simulink model "Flight_Physics__ForStudent"  (R2017b)
settings: configuration reference "cs" (kept outside this file)
undefined symbols (not defined in the file or in its folder): Actuators, AeroDerivatives, Configuration, Engine, g, magnitude, Sim_Control, Ts
libraries: aerolibatmos2 x1
settings Model: Creator=zht  LastModifiedBy=ZHT
settings ConfigSetRef: SourceLocation=Base Workspace

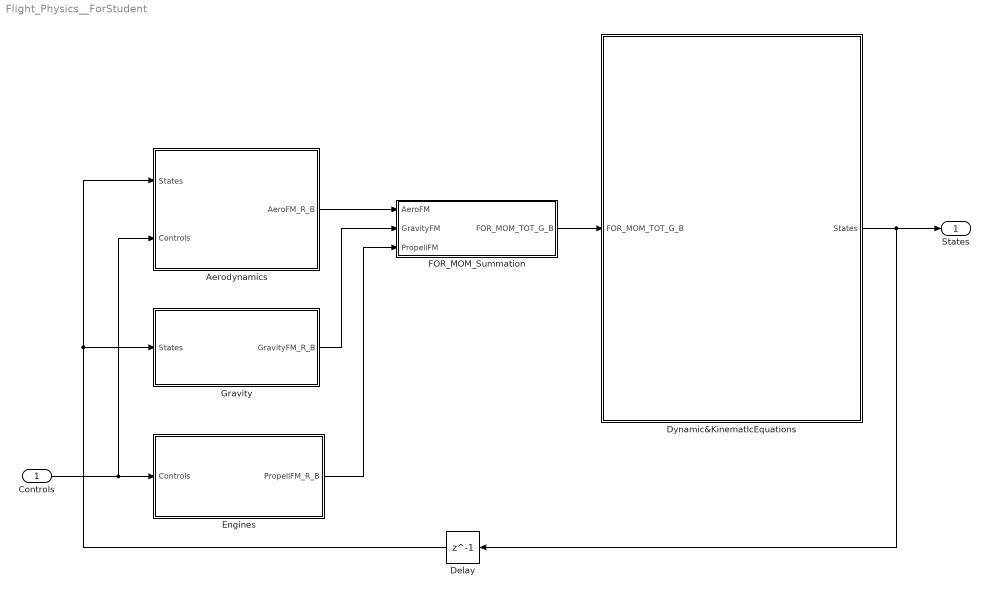
== system Flight_Physics__ForStudent ==
  Controls : Inport  OutDataTypeStr=Bus: Controls_CMD_BUS
  Aerodynamics : Subsystem
  Delay : Delay  DelayLength=1
  Dynamic&KinematlcEquations : Subsystem
  Engines : Subsystem
  FOR_MOM_Summation : Subsystem
  Gravity : Subsystem
  States : Outport  OutDataTypeStr=Bus: States_BUS
  wires:
  Controls/1 -> Engines/1(Controls), Aerodynamics/2(Controls)
  Dynamic&KinematlcEquations/1(States) -> States/1, Delay/1
  FOR_MOM_Summation/1(FOR_MOM_TOT_G_B) -> Dynamic&KinematlcEquations/1(FOR_MOM_TOT_G_B)
  Aerodynamics/1(AeroFM_R_B) -> FOR_MOM_Summation/1(AeroFM)
  Gravity/1(GravityFM_R_B) -> FOR_MOM_Summation/2(GravityFM)
  Engines/1(PropellFM_R_B) -> FOR_MOM_Summation/3(PropellFM)
  Delay/1 -> Aerodynamics/1(States), Gravity/1(States)

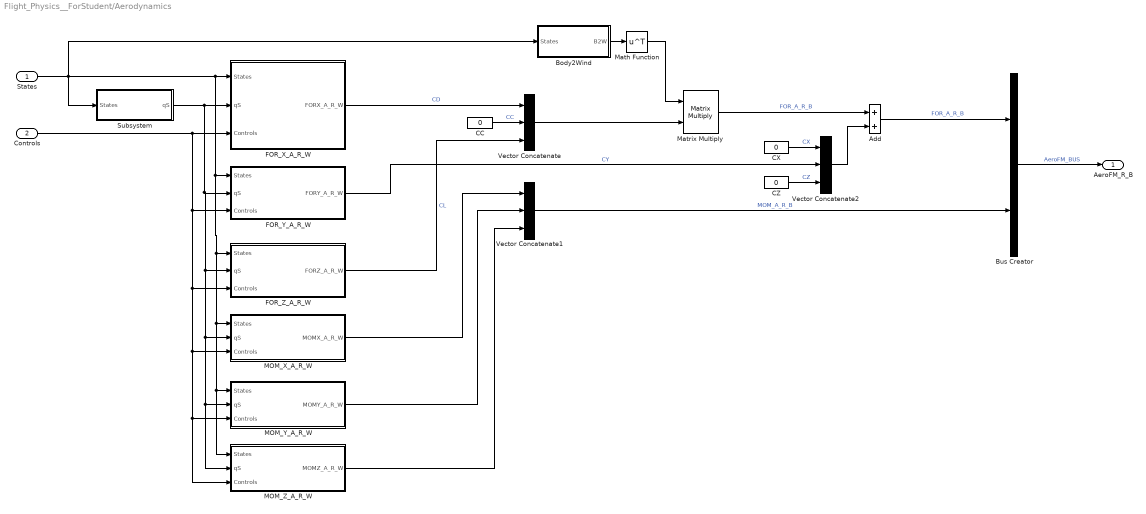
== system Flight_Physics__ForStudent/Aerodynamics ==
  States : Inport  OutDataTypeStr=Bus: States_BUS
  Controls : Inport  Port=2  OutDataTypeStr=Bus: Controls_CMD_BUS
  Add : Sum
  Body2Wind : Subsystem
  Bus Creator : BusCreator  Inputs=2  OutDataTypeStr=Bus: AeroFM_BUS
  CC : Constant  Value=0
  CX : Constant  Value=0
  CZ : Constant  Value=0
  FOR_X_A_R_W : Subsystem
  FOR_Y_A_R_W : Subsystem
  FOR_Z_A_R_W : Subsystem
  MOM_X_A_R_W : Subsystem
  MOM_Y_A_R_W : Subsystem
  MOM_Z_A_R_W : Subsystem
  Math Function : Math  Operator=transpose  SaturateOnIntegerOverflow=on
  Matrix Multiply : Product  Multiplication=Matrix(*)
  Subsystem : Subsystem
  Vector Concatenate : Concatenate  NumInputs=3  Mode=Multidimensional array
  Vector Concatenate1 : Concatenate  NumInputs=3  Mode=Multidimensional array
  Vector Concatenate2 : Concatenate  NumInputs=3  Mode=Multidimensional array
  AeroFM_R_B : Outport  OutDataTypeStr=Bus: AeroFM_BUS
  wires:
  Math Function/1 -> Matrix Multiply/1
  Add/1 -> Bus Creator/1  "FOR_A_R_B"
  Vector Concatenate1/1 -> Bus Creator/2  "MOM_A_R_B"
  MOM_Y_A_R_W/1(MOMY_A_R_W) -> Vector Concatenate1/2
  FOR_Z_A_R_W/1(FORZ_A_R_W) -> Vector Concatenate/3  "CL"
  FOR_Y_A_R_W/1(FORY_A_R_W) -> Vector Concatenate2/2  "CY"
  Body2Wind/1(B2W) -> Math Function/1
  Controls/1 -> FOR_Y_A_R_W/3(Controls), FOR_Z_A_R_W/3(Controls), MOM_X_A_R_W/3(Controls), MOM_Y_A_R_W/3(Controls), MOM_Z_A_R_W/3(Controls), FOR_X_A_R_W/3(Controls)
  Subsystem/1(qS) -> FOR_Z_A_R_W/2(qS), MOM_X_A_R_W/2(qS), MOM_Y_A_R_W/2(qS), MOM_Z_A_R_W/2(qS), FOR_Y_A_R_W/2(qS), FOR_X_A_R_W/2(qS)
  MOM_Z_A_R_W/1(MOMZ_A_R_W) -> Vector Concatenate1/3
  Bus Creator/1 -> AeroFM_R_B/1  "AeroFM_BUS"
  States/1 -> Subsystem/1(States), Body2Wind/1(States), MOM_Z_A_R_W/1(States), MOM_Y_A_R_W/1(States), MOM_X_A_R_W/1(States), FOR_Z_A_R_W/1(States), FOR_Y_A_R_W/1(States), FOR_X_A_R_W/1(States)
  MOM_X_A_R_W/1(MOMX_A_R_W) -> Vector Concatenate1/1
  FOR_X_A_R_W/1(FORX_A_R_W) -> Vector Concatenate/1  "CD"
  Vector Concatenate/1 -> Matrix Multiply/2
  CC/1 -> Vector Concatenate/2  "CC"
  CX/1 -> Vector Concatenate2/1  "CX"
  CZ/1 -> Vector Concatenate2/3  "CZ"
  Matrix Multiply/1 -> Add/1  "FOR_A_R_B"
  Vector Concatenate2/1 -> Add/2

== system Flight_Physics__ForStudent/Dynamic&KinematlcEquations ==
  note: 建模符号约定：
      | 变量命名：
      | 变量_运动类型_点_坐标系
      |
      | 变量类型：
      | VEL 速度（3x1的向量）
      | ROT 角速度（3x1的向量）
      | POS 位置（3x1的向量）
      | ATT 角度（3x1的向量）
      | VEL _DOT 加速度（3x1的向量）
      | ROT_DOT 角加速度（3x1的向量）
      | Alpha 迎角
      | Beta 侧滑角
      | Gamma 航迹倾角（下滑角、爬升角）
      | 运动类型：
      | K 表示相对于地面的运动
      | A 表示相对于气流的运动（考虑风场）
      | 点类型：
      | R 表示参考重心
      | G 表示实际重心
      | 坐标系类型：
      | B 机体系
      | E 地面系 ABS 与坐标系无关，表示该变量的绝对值
  FOR_MOM_TOT_G_B : Inport  OutDataTypeStr=Bus: FOR_MOM_TOT_BUS
  Bus Creator1 : BusCreator  Inputs=14  OutDataTypeStr=Bus: States_BUS
  Bus Selector1 : BusSelector  OutputSignals=FOR_T_G_B,MOM_T_G_B
  Bus Selector2 : BusSelector  OutputSignals=VEL_K_R_B,ROT_K_R_B,ATT_EULER
  Equations : Subsystem
  States : Outport  OutDataTypeStr=Bus: States_BUS
  wires:
  Bus Selector2/2 -> Equations/4(p_q_r)  "<ROT_K_R_B>"
  Bus Selector2/1 -> Equations/3(ub_vb_wb)  "<VEL_K_R_B>"
  Bus Selector2/3 -> Equations/5(phi_theta_psi)  "<ATT_EULER>"
  Equations/7(ROT_DOT_K_R_B) -> Bus Creator1/7  "ROT_DOT_K_R_B"
  Equations/10(VEL_K_R_ABS) -> Bus Creator1/10  "VEL_K_R_ABS"
  Bus Selector1/1 -> Equations/1(Fxyz(N))  "<FOR_T_G_B>"
  Equations/14(Beta_A_R_B) -> Bus Creator1/14  "Beta_A_R_B"
  Equations/12(Gamma_K_R_B) -> Bus Creator1/12  "Gamma_K_R_B"
  Equations/6(ROT_K_R_B) -> Bus Creator1/6  "ROT_K_R_B"
  Equations/13(Alpha_A_R_B) -> Bus Creator1/13  "Alpha_A_R_B"
  Equations/8(VEL_DOT_K_R_B) -> Bus Creator1/8  "VEL_DOT_K_R_B"
  Equations/5(VEL_K_R_B) -> Bus Creator1/5  "VEL_K_R_B"
  Equations/2(POS_R_E) -> Bus Creator1/2  "POS_R_E"
  Bus Creator1/1 -> Bus Selector2/1, States/1
  Bus Selector1/2 -> Equations/2(Mxyz(Nm))  "<MOM_T_G_B>"
  Equations/11(Chi_K_R_B) -> Bus Creator1/11  "Chi_K_R_B"
  Equations/1(VEL_K_R_E) -> Bus Creator1/1  "VEL_K_R_E"
  FOR_MOM_TOT_G_B/1 -> Bus Selector1/1
  Equations/9(FUEL_Availible) -> Bus Creator1/9  "FUEL_Availible"
  Equations/3(ATT_EULER) -> Bus Creator1/3  "ATT_EULER"
  Equations/4(M_BE) -> Bus Creator1/4  "M_BE"

== system Flight_Physics__ForStudent/Engines ==
  Controls : Inport  OutDataTypeStr=Bus: Controls_CMD_BUS
  1-D Lookup Table : Lookup_n-D  NumberOfTableDimensions=1  BreakpointsForDimension1=Engine.Thrset  Table=Engine.Tset  InternalRulePriority=Speed  RndMeth=Simplest  InputSameDT=on
  1-D Lookup Table1 : Lookup_n-D  NumberOfTableDimensions=1  BreakpointsForDimension1=Engine.Thrset  Table=Engine.SFCset  InternalRulePriority=Speed  RndMeth=Simplest  InputSameDT=on
  Bus Creator : BusCreator  Inputs=3  OutDataTypeStr=Bus: PropellFM_BUS
  Bus Selector : BusSelector  OutputSignals=Engine_CMD
  Constant4 : Constant  Value=Engine.Position-Configuration.POS_CG  SampleTime=Ts
  Constant5 : Constant  Value=Engine.Phi  SampleTime=Ts
  Gain : Gain  Gain=[1,0,0]'
  Gain1 : Gain  Gain=100
  Matrix Multiply : Product  Multiplication=Matrix(*)
  Subsystem : Subsystem
  Subsystem1 : Subsystem
  PropellFM_R_B : Outport  OutDataTypeStr=Bus: PropellFM_BUS
  wires:
  1-D Lookup Table1/1 -> Bus Creator/3  "SFC"
  Subsystem/1(M_B_Phi) -> Matrix Multiply/1
  Matrix Multiply/1 -> Subsystem1/2(v2), Bus Creator/2  "FOR_P_R_B"
  Bus Creator/1 -> PropellFM_R_B/1  "PropellFM_BUS"
  Bus Selector/1 -> 1-D Lookup Table1/1, Gain1/1  "<Engine_CMD>"
  Gain1/1 -> 1-D Lookup Table/1
  1-D Lookup Table/1 -> Gain/1
  Constant4/1 -> Subsystem1/1(v1)
  Controls/1 -> Bus Selector/1
  Gain/1 -> Matrix Multiply/2
  Constant5/1 -> Subsystem/1(Phi_rad)
  Subsystem1/1(v1_x_v2) -> Bus Creator/1  "MOM_P_R_B"

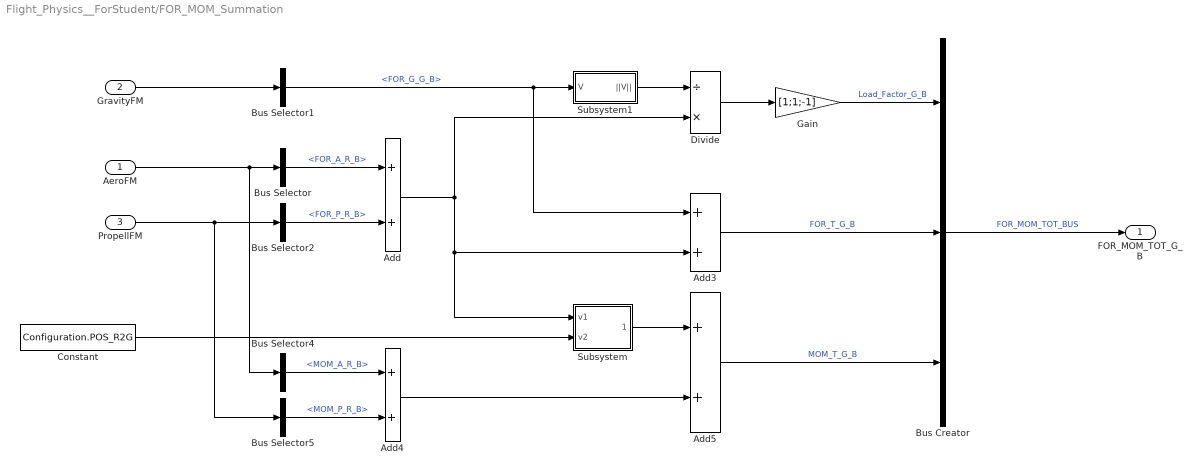
== system Flight_Physics__ForStudent/FOR_MOM_Summation ==
  AeroFM : Inport  OutDataTypeStr=Bus: AeroFM_BUS
  GravityFM : Inport  Port=2  OutDataTypeStr=Bus: GravityFM_BUS
  PropellFM : Inport  Port=3  OutDataTypeStr=Bus: PropellFM_BUS
  Add{,3..5} (4 alike) : Sum
  Bus Creator : BusCreator  Inputs=3  OutDataTypeStr=Bus: FOR_MOM_TOT_BUS
  Bus Selector : BusSelector  OutputSignals=FOR_A_R_B
  Bus Selector1 : BusSelector  OutputSignals=FOR_G_G_B
  Bus Selector2 : BusSelector  OutputSignals=FOR_P_R_B
  Bus Selector4 : BusSelector  OutputSignals=MOM_A_R_B
  Bus Selector5 : BusSelector  OutputSignals=MOM_P_R_B
  Constant : Constant  Value=Configuration.POS_R2G
  Divide : Product  Inputs=/*
  Gain : Gain  Gain=[1;1;-1]
  Subsystem : Subsystem
  Subsystem1 : Subsystem
  FOR_MOM_TOT_G_B : Outport  OutDataTypeStr=Bus: FOR_MOM_TOT_BUS
  wires:
  PropellFM/1 -> Bus Selector2/1, Bus Selector5/1
  AeroFM/1 -> Bus Selector4/1, Bus Selector/1
  GravityFM/1 -> Bus Selector1/1
  Bus Creator/1 -> FOR_MOM_TOT_G_B/1  "FOR_MOM_TOT_BUS"
  Bus Selector/1 -> Add/1  "<FOR_A_R_B>"
  Bus Selector2/1 -> Add/2  "<FOR_P_R_B>"
  Bus Selector1/1 -> Subsystem1/1(V), Add3/1  "<FOR_G_G_B>"
  Add/1 -> Subsystem/1(v1), Add3/2, Divide/2
  Subsystem1/1(||V||) -> Divide/1
  Divide/1 -> Gain/1
  Gain/1 -> Bus Creator/1  "Load_Factor_G_B"
  Add3/1 -> Bus Creator/2  "FOR_T_G_B"
  Bus Selector4/1 -> Add4/1  "<MOM_A_R_B>"
  Bus Selector5/1 -> Add4/2  "<MOM_P_R_B>"
  Subsystem/1(v1_x_v2) -> Add5/1
  Add4/1 -> Add5/2
  Add5/1 -> Bus Creator/3  "MOM_T_G_B"
  Constant/1 -> Subsystem/2(v2)

== system Flight_Physics__ForStudent/Gravity ==
  States : Inport  OutDataTypeStr=Bus: States_BUS
  Bus Creator : BusCreator  Inputs=2  OutDataTypeStr=Bus: GravityFM_BUS
  Bus Selector : BusSelector  OutputSignals=M_BE
  Constant : Constant  Value=[0;0;0]
  Constant1 : Constant  Value=[0;0;g]  SampleTime=Ts
  Constant2 : Constant  Value=Configuration.Mass  SampleTime=Ts
  Matrix Multiply : Product  Multiplication=Matrix(*)
  Product : Product
  GravityFM_R_B : Outport  OutDataTypeStr=Bus: GravityFM_BUS
  wires:
  States/1 -> Bus Selector/1
  Bus Selector/1 -> Matrix Multiply/1  "<M_BE>"
  Constant1/1 -> Matrix Multiply/2
  Matrix Multiply/1 -> Product/1
  Constant2/1 -> Product/2
  Product/1 -> Bus Creator/1  "FOR_G_G_B"
  Constant/1 -> Bus Creator/2  "MOM_G_G_B"
  Bus Creator/1 -> GravityFM_R_B/1  "GravityFM_BUS"

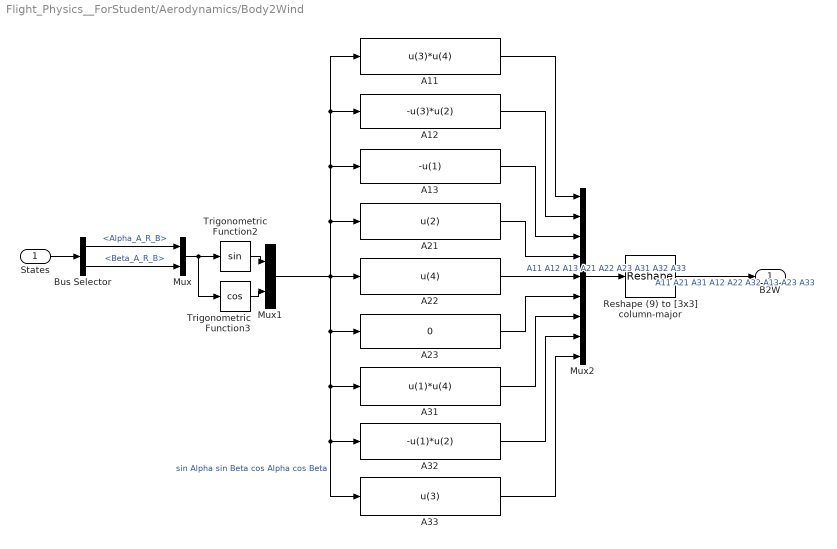
== system Flight_Physics__ForStudent/Aerodynamics/Body2Wind ==
  States : Inport  OutDataTypeStr=Bus: States_BUS
  A11 : Fcn  Expr=u(3)*u(4)
  A12 : Fcn  Expr=-u(3)*u(2)
  A13 : Fcn  Expr=-u(1)
  A21 : Fcn  Expr=u(2)
  A22 : Fcn  Expr=u(4)
  A23 : Fcn  Expr=0
  A31 : Fcn  Expr=u(1)*u(4)
  A32 : Fcn  Expr=-u(1)*u(2)
  A33 : Fcn  Expr=u(3)
  Bus Selector : BusSelector  OutputSignals=Alpha_A_R_B,Beta_A_R_B
  Mux : Mux  Inputs=2
  Mux1 : Mux  Inputs=2
  Mux2 : Mux  Inputs=9
  Reshape (9) to [3x3] column-major : Reshape  OutputDimensionality=Customize  OutputDimensions=[3,3]
  Trigonometric Function2 : Trigonometry
  Trigonometric Function3 : Trigonometry  Operator=cos
  B2W : Outport  PortDimensions=[3 3]
  wires:
  Mux/1 -> Trigonometric Function2/1, Trigonometric Function3/1
  Trigonometric Function3/1 -> Mux1/2
  Trigonometric Function2/1 -> Mux1/1
  Bus Selector/2 -> Mux/2  "<Beta_A_R_B>"
  Bus Selector/1 -> Mux/1  "<Alpha_A_R_B>"
  States/1 -> Bus Selector/1
  A12/1 -> Mux2/2
  A13/1 -> Mux2/3
  A21/1 -> Mux2/4
  A32/1 -> Mux2/8
  A23/1 -> Mux2/6
  Mux2/1 -> Reshape (9) to [3x3] column-major/1  "A11 A12 A13 A21 A22 A23 A31 A32 A33"
  Reshape (9) to [3x3] column-major/1 -> B2W/1  "A11 A21 A31 A12 A22 A32 A13 A23 A33"
  A11/1 -> Mux2/1
  A22/1 -> Mux2/5
  A33/1 -> Mux2/9
  Mux1/1 -> A22/1, A23/1, A31/1, A32/1, A33/1, A21/1, A13/1, A11/1, A12/1  "sin Alpha sin Beta cos Alpha cos Beta"
  A31/1 -> Mux2/7

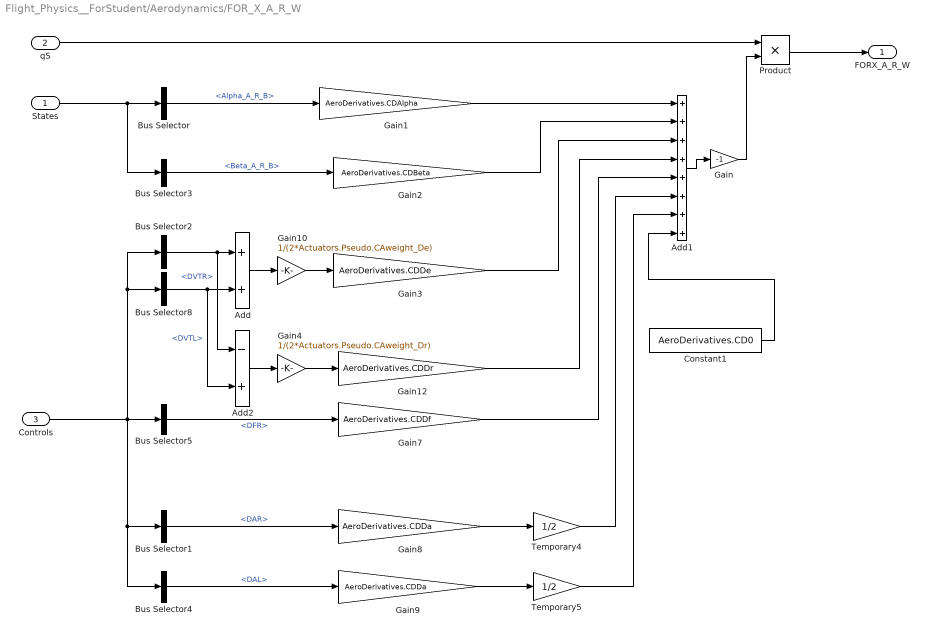
== system Flight_Physics__ForStudent/Aerodynamics/FOR_X_A_R_W ==
  States : Inport  OutDataTypeStr=Bus: States_BUS  BusOutputAsStruct=on
  qS : Inport  Port=2  BusOutputAsStruct=on
  Controls : Inport  Port=3  OutDataTypeStr=Bus: Controls_CMD_BUS  BusOutputAsStruct=on
  Add : Sum
  Add1 : Sum  Inputs=++++++++
  Add2 : Sum  Inputs=-+
  Bus Selector : BusSelector  OutputSignals=Alpha_A_R_B
  Bus Selector1 : BusSelector  OutputSignals=Actuators_CMD.DAR
  Bus Selector2 : BusSelector  OutputSignals=Actuators_CMD.DVTR
  Bus Selector3 : BusSelector  OutputSignals=Beta_A_R_B
  Bus Selector4 : BusSelector  OutputSignals=Actuators_CMD.DAL
  Bus Selector5 : BusSelector  OutputSignals=Actuators_CMD.DFR
  Bus Selector8 : BusSelector  OutputSignals=Actuators_CMD.DVTL
  Constant1 : Constant  Value=AeroDerivatives.CD0
  Gain : Gain  Gain=-1
  Gain1 : Gain  Gain=AeroDerivatives.CDAlpha
  Gain10 : Gain  Gain=1/(2*Actuators.Pseudo.CAweight_De)
  Gain12 : Gain  Gain=AeroDerivatives.CDDr
  Gain2 : Gain  Gain=AeroDerivatives.CDBeta
  Gain3 : Gain  Gain=AeroDerivatives.CDDe
  Gain4 : Gain  Gain=1/(2*Actuators.Pseudo.CAweight_Dr)
  Gain7 : Gain  Gain=AeroDerivatives.CDDf
  Gain8 : Gain  Gain=AeroDerivatives.CDDa
  Gain9 : Gain  Gain=AeroDerivatives.CDDa
  Product : Product
  Temporary4 : Gain  Gain=1/2
  Temporary5 : Gain  Gain=1/2
  FORX_A_R_W : Outport  Unit=N  PortDimensions=1
  wires:
  Bus Selector2/1 -> Add2/1, Add/1  "<DVTR>"
  Bus Selector8/1 -> Add2/2, Add/2  "<DVTL>"
  Gain2/1 -> Add1/2
  Product/1 -> FORX_A_R_W/1
  Controls/1 -> Bus Selector5/1, Bus Selector1/1, Bus Selector4/1, Bus Selector2/1, Bus Selector8/1
  Gain1/1 -> Add1/1
  Gain3/1 -> Add1/3
  Gain/1 -> Product/2
  Gain4/1 -> Gain12/1
  States/1 -> Bus Selector3/1, Bus Selector/1
  Bus Selector5/1 -> Gain7/1  "<DFR>"
  Bus Selector/1 -> Gain1/1  "<Alpha_A_R_B>"
  Add1/1 -> Gain/1
  Bus Selector3/1 -> Gain2/1  "<Beta_A_R_B>"
  Bus Selector1/1 -> Gain8/1  "<DAR>"
  Bus Selector4/1 -> Gain9/1  "<DAL>"
  Gain8/1 -> Temporary4/1
  Gain9/1 -> Temporary5/1
  qS/1 -> Product/1
  Add/1 -> Gain10/1
  Gain10/1 -> Gain3/1
  Add2/1 -> Gain4/1
  Gain12/1 -> Add1/4
  Gain7/1 -> Add1/5
  Temporary4/1 -> Add1/6
  Temporary5/1 -> Add1/7
  Constant1/1 -> Add1/8

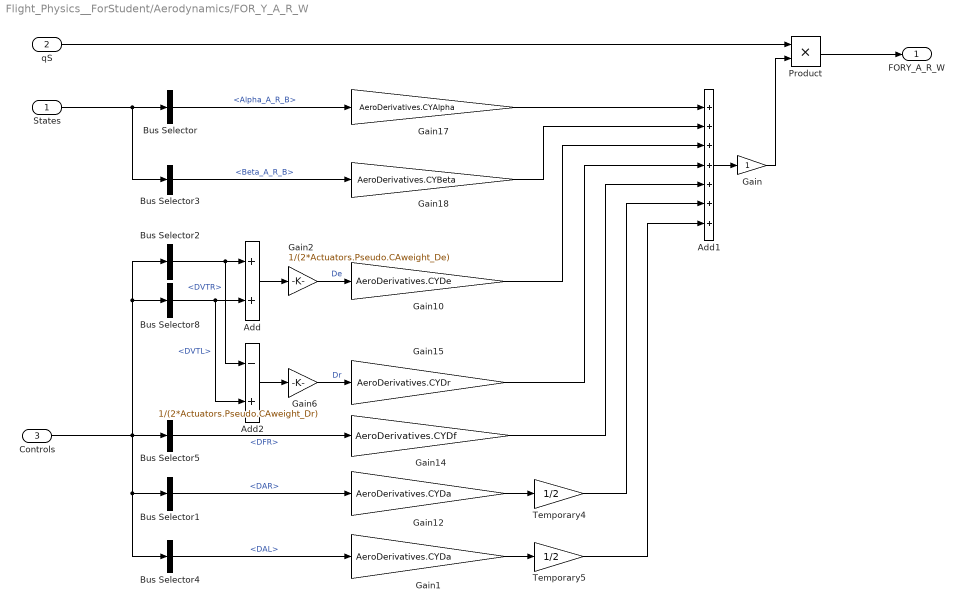
== system Flight_Physics__ForStudent/Aerodynamics/FOR_Y_A_R_W ==
  States : Inport  OutDataTypeStr=Bus: States_BUS  BusOutputAsStruct=on
  qS : Inport  Port=2  BusOutputAsStruct=on
  Controls : Inport  Port=3  OutDataTypeStr=Bus: Controls_CMD_BUS  BusOutputAsStruct=on
  Add : Sum
  Add1 : Sum  Inputs=+++++++
  Add2 : Sum  Inputs=-+
  Bus Selector : BusSelector  OutputSignals=Alpha_A_R_B
  Bus Selector1 : BusSelector  OutputSignals=Actuators_CMD.DAR
  Bus Selector2 : BusSelector  OutputSignals=Actuators_CMD.DVTR
  Bus Selector3 : BusSelector  OutputSignals=Beta_A_R_B
  Bus Selector4 : BusSelector  OutputSignals=Actuators_CMD.DAL
  Bus Selector5 : BusSelector  OutputSignals=Actuators_CMD.DFR
  Bus Selector8 : BusSelector  OutputSignals=Actuators_CMD.DVTL
  Gain : Gain
  Gain1 : Gain  Gain=AeroDerivatives.CYDa
  Gain10 : Gain  Gain=AeroDerivatives.CYDe
  Gain12 : Gain  Gain=AeroDerivatives.CYDa
  Gain14 : Gain  Gain=AeroDerivatives.CYDf
  Gain15 : Gain  Gain=AeroDerivatives.CYDr
  Gain17 : Gain  Gain=AeroDerivatives.CYAlpha
  Gain18 : Gain  Gain=AeroDerivatives.CYBeta
  Gain2 : Gain  Gain=1/(2*Actuators.Pseudo.CAweight_De)
  Gain6 : Gain  Gain=1/(2*Actuators.Pseudo.CAweight_Dr)
  Product : Product
  Temporary4 : Gain  Gain=1/2
  Temporary5 : Gain  Gain=1/2
  FORY_A_R_W : Outport  Unit=N  PortDimensions=1
  wires:
  Bus Selector3/1 -> Gain18/1  "<Beta_A_R_B>"
  Gain12/1 -> Temporary4/1
  Gain18/1 -> Add1/2
  Gain2/1 -> Gain10/1  "De"
  qS/1 -> Product/1
  States/1 -> Bus Selector3/1, Bus Selector/1
  Add1/1 -> Gain/1
  Controls/1 -> Bus Selector5/1, Bus Selector1/1, Bus Selector4/1, Bus Selector2/1, Bus Selector8/1
  Bus Selector1/1 -> Gain12/1  "<DAR>"
  Gain1/1 -> Temporary5/1
  Gain/1 -> Product/2
  Bus Selector2/1 -> Add2/1, Add/1  "<DVTR>"
  Bus Selector/1 -> Gain17/1  "<Alpha_A_R_B>"
  Bus Selector5/1 -> Gain14/1  "<DFR>"
  Temporary5/1 -> Add1/7
  Temporary4/1 -> Add1/6
  Product/1 -> FORY_A_R_W/1
  Bus Selector4/1 -> Gain1/1  "<DAL>"
  Gain17/1 -> Add1/1
  Gain14/1 -> Add1/5
  Gain6/1 -> Gain15/1  "Dr"
  Gain15/1 -> Add1/4
  Add2/1 -> Gain6/1
  Bus Selector8/1 -> Add2/2, Add/2  "<DVTL>"
  Add/1 -> Gain2/1
  Gain10/1 -> Add1/3

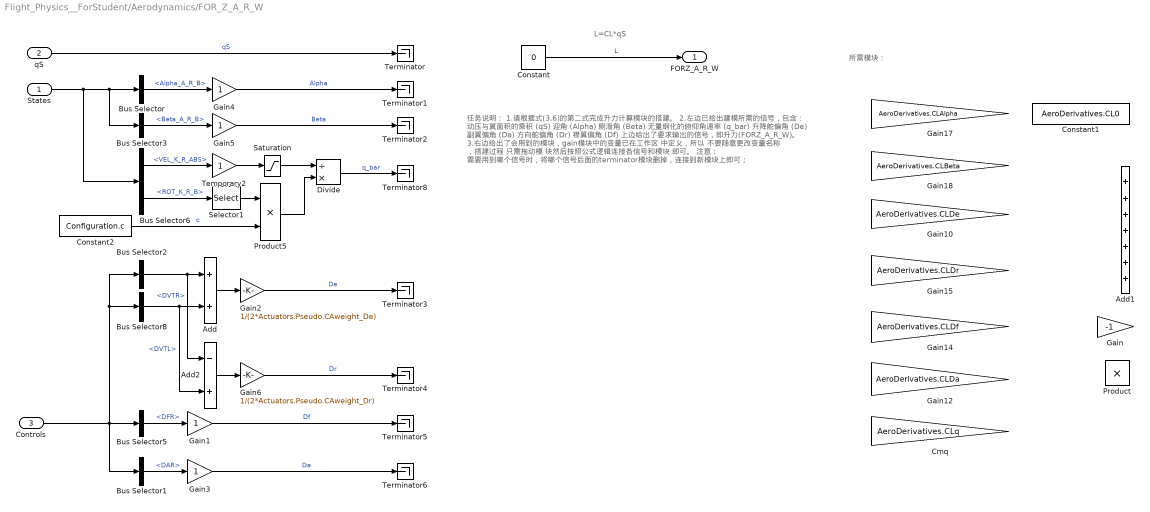
== system Flight_Physics__ForStudent/Aerodynamics/FOR_Z_A_R_W ==
  note: L=CL*qS
  note: 任务说明：
      |
      | 1.请根据式(3.6)的第二式完成升力计算模块的搭建。
      |
      | 2.左边已给出建模所需的信号，包含：
      |
      | 动压与翼面积的乘积 (qS)
      |
      | 迎角 (Alpha)
      |
      | 侧滑角 (Beta)
      |
      | 无量纲化的俯仰角速率 (q_bar)
      |
      | 升降舵偏角 (De)
      |
      | 副翼偏角 (Da)
      |
      | 方向舵偏角 (Dr)
      |
      | 襟翼偏角 (Df)
      |
      | 上边给出了要求输出的信号，即升力(FORZ_A_R_W)。
      |
      | 3.右边给出了会用到的模块，gain模块中的变量已在工作区
      |
      | 中定义，所以 不要随意更改变量名称 ，搭建过程 只需拖动模
      |
      | 块然后按照公式逻辑连接各信号和模块 即可。
      |
      | 注意：
      |
      | 需要用到哪个信号时，将哪个信号后面的terminator模块删掉，连接到新模块上即可；
  note: 所需模块：
  States : Inport  OutDataTypeStr=Bus: States_BUS  BusOutputAsStruct=on
  qS : Inport  Port=2  BusOutputAsStruct=on
  Controls : Inport  Port=3  OutDataTypeStr=Bus: Controls_CMD_BUS  BusOutputAsStruct=on
  Add : Sum
  Add1 : Sum  Inputs=+++++++
  Add2 : Sum  Inputs=-+
  Bus Selector : BusSelector  OutputSignals=Alpha_A_R_B
  Bus Selector1 : BusSelector  OutputSignals=Actuators_CMD.DAR
  Bus Selector2 : BusSelector  OutputSignals=Actuators_CMD.DVTR
  Bus Selector3 : BusSelector  OutputSignals=Beta_A_R_B
  Bus Selector5 : BusSelector  OutputSignals=Actuators_CMD.DFR
  Bus Selector6 : BusSelector  OutputSignals=VEL_K_R_ABS,ROT_K_R_B
  Bus Selector8 : BusSelector  OutputSignals=Actuators_CMD.DVTL
  Cmq : Gain  Gain=AeroDerivatives.CLq
  Constant : Constant  Value=0
  Constant1 : Constant  Value=AeroDerivatives.CL0
  Constant2 : Constant  Value=Configuration.c
  Divide : Product  Inputs=/*
  Gain : Gain  Gain=-1
  Gain{1,3..5} (4 alike) : Gain
  Gain10 : Gain  Gain=AeroDerivatives.CLDe
  Gain12 : Gain  Gain=AeroDerivatives.CLDa
  Gain14 : Gain  Gain=AeroDerivatives.CLDf
  Gain15 : Gain  Gain=AeroDerivatives.CLDr
  Gain17 : Gain  Gain=AeroDerivatives.CLAlpha
  Gain18 : Gain  Gain=AeroDerivatives.CLBeta
  Gain2 : Gain  Gain=1/(2*Actuators.Pseudo.CAweight_De)
  Gain6 : Gain  Gain=1/(2*Actuators.Pseudo.CAweight_Dr)
  Product : Product
  Product5 : Product
  Saturation : Saturate  UpperLimit=inf  LowerLimit=10
  Selector1 : Selector  InputPortWidth=3  IndexOptions=Index vector (dialog)  Indices=[2]  OutputSizes=1
  Temporary2 : Gain
  Terminator{,1..6,8} (8 alike) : Terminator
  FORZ_A_R_W : Outport  Unit=N  PortDimensions=1
  wires:
  Add/1 -> Gain2/1
  Bus Selector8/1 -> Add/2, Add2/2  "<DVTL>"
  Add2/1 -> Gain6/1
  Gain6/1 -> Terminator4/1  "Dr"
  Bus Selector5/1 -> Gain1/1  "<DFR>"
  Bus Selector/1 -> Gain4/1  "<Alpha_A_R_B>"
  Bus Selector2/1 -> Add/1, Add2/1  "<DVTR>"
  Bus Selector1/1 -> Gain3/1  "<DAR>"
  Controls/1 -> Bus Selector8/1, Bus Selector2/1, Bus Selector1/1, Bus Selector5/1
  States/1 -> Bus Selector6/1, Bus Selector/1, Bus Selector3/1
  Gain2/1 -> Terminator3/1  "De"
  Bus Selector3/1 -> Gain5/1  "<Beta_A_R_B>"
  qS/1 -> Terminator/1  "qS"
  Constant/1 -> FORZ_A_R_W/1  "L"
  Gain1/1 -> Terminator5/1  "Df"
  Gain3/1 -> Terminator6/1  "Da"
  Gain4/1 -> Terminator1/1  "Alpha"
  Gain5/1 -> Terminator2/1  "Beta"
  Constant2/1 -> Product5/2  "c"
  Temporary2/1 -> Saturation/1
  Saturation/1 -> Divide/1
  Bus Selector6/1 -> Temporary2/1  "<VEL_K_R_ABS>"
  Divide/1 -> Terminator8/1  "q_bar"
  Selector1/1 -> Product5/1
  Bus Selector6/2 -> Selector1/1  "<ROT_K_R_B>"
  Product5/1 -> Divide/2

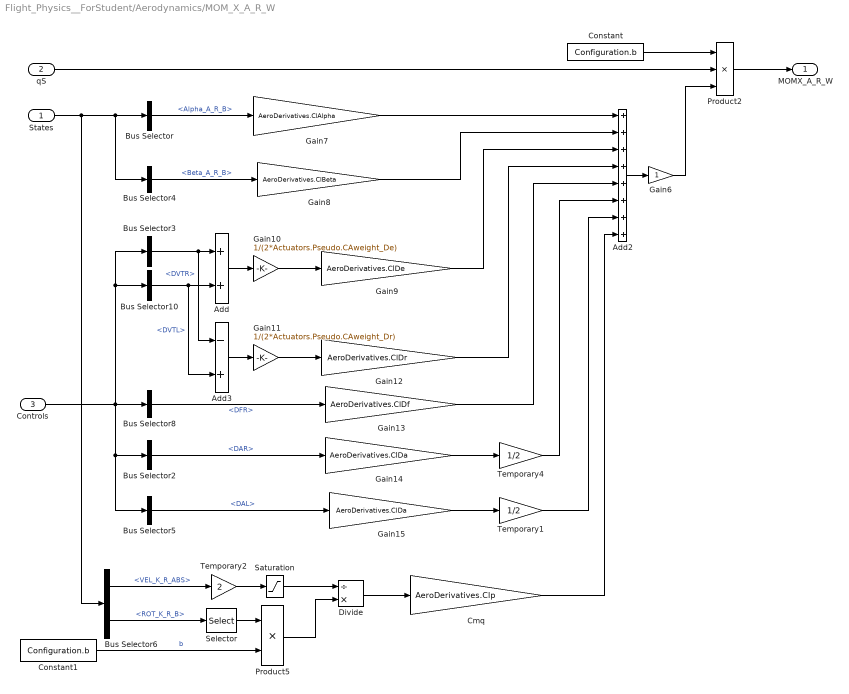
== system Flight_Physics__ForStudent/Aerodynamics/MOM_X_A_R_W ==
  States : Inport  OutDataTypeStr=Bus: States_BUS  BusOutputAsStruct=on
  qS : Inport  Port=2  BusOutputAsStruct=on
  Controls : Inport  Port=3  OutDataTypeStr=Bus: Controls_CMD_BUS  BusOutputAsStruct=on
  Add : Sum
  Add2 : Sum  Inputs=++++++++
  Add3 : Sum  Inputs=-+
  Bus Selector : BusSelector  OutputSignals=Alpha_A_R_B
  Bus Selector10 : BusSelector  OutputSignals=Actuators_CMD.DVTL
  Bus Selector2 : BusSelector  OutputSignals=Actuators_CMD.DAR
  Bus Selector3 : BusSelector  OutputSignals=Actuators_CMD.DVTR
  Bus Selector4 : BusSelector  OutputSignals=Beta_A_R_B
  Bus Selector5 : BusSelector  OutputSignals=Actuators_CMD.DAL
  Bus Selector6 : BusSelector  OutputSignals=VEL_K_R_ABS,ROT_K_R_B
  Bus Selector8 : BusSelector  OutputSignals=Actuators_CMD.DFR
  Cmq : Gain  Gain=AeroDerivatives.Clp
  Constant : Constant  Value=Configuration.b
  Constant1 : Constant  Value=Configuration.b
  Divide : Product  Inputs=/*
  Gain10 : Gain  Gain=1/(2*Actuators.Pseudo.CAweight_De)
  Gain11 : Gain  Gain=1/(2*Actuators.Pseudo.CAweight_Dr)
  Gain12 : Gain  Gain=AeroDerivatives.ClDr
  Gain13 : Gain  Gain=AeroDerivatives.ClDf
  Gain14 : Gain  Gain=AeroDerivatives.ClDa
  Gain15 : Gain  Gain=AeroDerivatives.ClDa
  Gain6 : Gain
  Gain7 : Gain  Gain=AeroDerivatives.ClAlpha
  Gain8 : Gain  Gain=AeroDerivatives.ClBeta
  Gain9 : Gain  Gain=AeroDerivatives.ClDe
  Product2 : Product  Inputs=3
  Product5 : Product
  Saturation : Saturate  UpperLimit=inf  LowerLimit=10
  Selector : Selector  InputPortWidth=3  IndexOptions=Index vector (dialog)  Indices=[1]  OutputSizes=1
  Temporary1 : Gain  Gain=1/2
  Temporary2 : Gain  Gain=2
  Temporary4 : Gain  Gain=1/2
  MOMX_A_R_W : Outport  Unit=N  PortDimensions=1
  wires:
  Bus Selector4/1 -> Gain8/1  "<Beta_A_R_B>"
  Gain14/1 -> Temporary4/1
  Gain8/1 -> Add2/2
  Gain10/1 -> Gain9/1
  qS/1 -> Product2/2
  States/1 -> Bus Selector6/1, Bus Selector4/1, Bus Selector/1
  Add2/1 -> Gain6/1
  Controls/1 -> Bus Selector8/1, Bus Selector2/1, Bus Selector5/1, Bus Selector3/1, Bus Selector10/1
  Bus Selector2/1 -> Gain14/1  "<DAR>"
  Gain15/1 -> Temporary1/1
  Gain6/1 -> Product2/3
  Bus Selector3/1 -> Add3/1, Add/1  "<DVTR>"
  Bus Selector/1 -> Gain7/1  "<Alpha_A_R_B>"
  Bus Selector8/1 -> Gain13/1  "<DFR>"
  Temporary1/1 -> Add2/7
  Temporary4/1 -> Add2/6
  Product2/1 -> MOMX_A_R_W/1
  Bus Selector5/1 -> Gain15/1  "<DAL>"
  Gain7/1 -> Add2/1
  Gain13/1 -> Add2/5
  Gain11/1 -> Gain12/1
  Gain12/1 -> Add2/4
  Add3/1 -> Gain11/1
  Bus Selector10/1 -> Add3/2, Add/2  "<DVTL>"
  Add/1 -> Gain10/1
  Gain9/1 -> Add2/3
  Constant/1 -> Product2/1
  Product5/1 -> Divide/2
  Saturation/1 -> Divide/1
  Constant1/1 -> Product5/2  "b"
  Selector/1 -> Product5/1
  Temporary2/1 -> Saturation/1
  Divide/1 -> Cmq/1
  Bus Selector6/1 -> Temporary2/1  "<VEL_K_R_ABS>"
  Bus Selector6/2 -> Selector/1  "<ROT_K_R_B>"
  Cmq/1 -> Add2/8

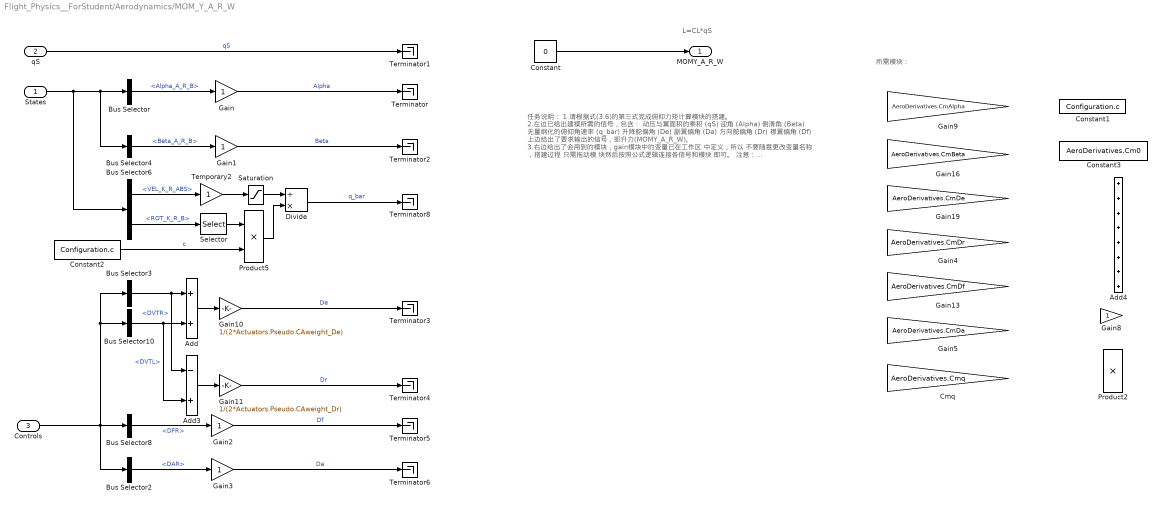
== system Flight_Physics__ForStudent/Aerodynamics/MOM_Y_A_R_W ==
  note: 所需模块：
  note: 任务说明：
      |
      | 1.请根据式(3.6)的第三式完成俯仰力矩计算模块的搭建。
      |
      | 2.左边已给出建模所需的信号，包含：
      |
      | 动压与翼面积的乘积 (qS)
      |
      | 迎角 (Alpha)
      |
      | 侧滑角 (Beta)
      |
      | 无量纲化的俯仰角速率 (q_bar)
      |
      | 升降舵偏角 (De)
      |
      | 副翼偏角 (Da)
      |
      | 方向舵偏角 (Dr)
      |
      | 襟翼偏角 (Df)
      |
      | 上边给出了要求输出的信号，即升力(MOMY_A_R_W)。
      |
      | 3.右边给出了会用到的模块，gain模块中的变量已在工作区
      |
      | 中定义，所以 不要随意更改变量名称 ，搭建过程 只需拖动模
      |
      | 块然后按照公式逻辑连接各信号和模块 即可。
      |
      | 注意：
      |
      | 需要用到哪个信号时，将哪个信号后面的terminator模块删掉，连接到新模块上即可；
  note: L=CL*qS
  States : Inport  OutDataTypeStr=Bus: States_BUS  BusOutputAsStruct=on
  qS : Inport  Port=2  BusOutputAsStruct=on
  Controls : Inport  Port=3  OutDataTypeStr=Bus: Controls_CMD_BUS  BusOutputAsStruct=on
  Add : Sum
  Add3 : Sum  Inputs=-+
  Add4 : Sum  Inputs=++++++++
  Bus Selector : BusSelector  OutputSignals=Alpha_A_R_B
  Bus Selector10 : BusSelector  OutputSignals=Actuators_CMD.DVTL
  Bus Selector2 : BusSelector  OutputSignals=Actuators_CMD.DAR
  Bus Selector3 : BusSelector  OutputSignals=Actuators_CMD.DVTR
  Bus Selector4 : BusSelector  OutputSignals=Beta_A_R_B
  Bus Selector6 : BusSelector  OutputSignals=VEL_K_R_ABS,ROT_K_R_B
  Bus Selector8 : BusSelector  OutputSignals=Actuators_CMD.DFR
  Cmq : Gain  Gain=AeroDerivatives.Cmq
  Constant : Constant  Value=0
  Constant1 : Constant  Value=Configuration.c
  Constant2 : Constant  Value=Configuration.c
  Constant3 : Constant  Value=AeroDerivatives.Cm0
  Divide : Product  Inputs=/*
  Gain{,1..3,8} (5 alike) : Gain
  Gain10 : Gain  Gain=1/(2*Actuators.Pseudo.CAweight_De)
  Gain11 : Gain  Gain=1/(2*Actuators.Pseudo.CAweight_Dr)
  Gain13 : Gain  Gain=AeroDerivatives.CmDf
  Gain16 : Gain  Gain=AeroDerivatives.CmBeta
  Gain19 : Gain  Gain=AeroDerivatives.CmDe
  Gain4 : Gain  Gain=AeroDerivatives.CmDr
  Gain5 : Gain  Gain=AeroDerivatives.CmDa
  Gain9 : Gain  Gain=AeroDerivatives.CmAlpha
  Product2 : Product  Inputs=3
  Product5 : Product
  Saturation : Saturate  UpperLimit=inf  LowerLimit=10
  Selector : Selector  InputPortWidth=3  IndexOptions=Index vector (dialog)  Indices=[2]  OutputSizes=1
  Temporary2 : Gain
  Terminator{,1..6,8} (8 alike) : Terminator
  MOMY_A_R_W : Outport  Unit=N  PortDimensions=1
  wires:
  Add/1 -> Gain10/1
  Bus Selector10/1 -> Add/2, Add3/2  "<DVTL>"
  Add3/1 -> Gain11/1
  Gain11/1 -> Terminator4/1  "Dr"
  Bus Selector8/1 -> Gain2/1  "<DFR>"
  Bus Selector/1 -> Gain/1  "<Alpha_A_R_B>"
  Bus Selector3/1 -> Add/1, Add3/1  "<DVTR>"
  Bus Selector2/1 -> Gain3/1  "<DAR>"
  Controls/1 -> Bus Selector10/1, Bus Selector3/1, Bus Selector2/1, Bus Selector8/1
  Gain10/1 -> Terminator3/1  "De"
  Bus Selector4/1 -> Gain1/1  "<Beta_A_R_B>"
  Temporary2/1 -> Saturation/1
  Selector/1 -> Product5/1
  Product5/1 -> Divide/2
  Bus Selector6/2 -> Selector/1  "<ROT_K_R_B>"
  Saturation/1 -> Divide/1
  Bus Selector6/1 -> Temporary2/1  "<VEL_K_R_ABS>"
  States/1 -> Bus Selector6/1, Bus Selector/1, Bus Selector4/1
  Constant2/1 -> Product5/2  "c"
  qS/1 -> Terminator1/1  "qS"
  Divide/1 -> Terminator8/1  "q_bar"
  Gain/1 -> Terminator/1  "Alpha"
  Gain1/1 -> Terminator2/1  "Beta"
  Gain2/1 -> Terminator5/1  "Df"
  Gain3/1 -> Terminator6/1  "Da"
  Constant/1 -> MOMY_A_R_W/1

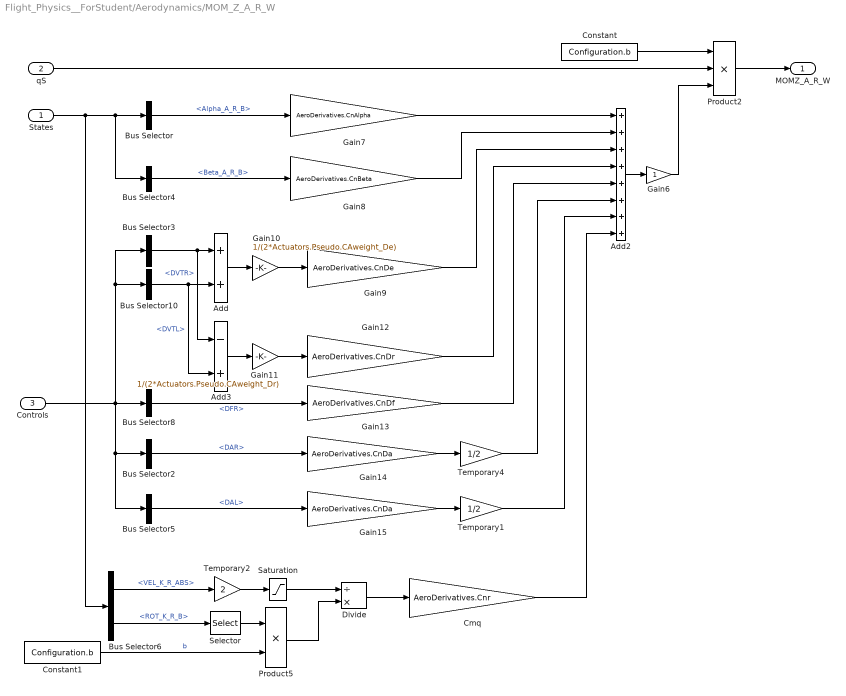
== system Flight_Physics__ForStudent/Aerodynamics/MOM_Z_A_R_W ==
  States : Inport  OutDataTypeStr=Bus: States_BUS  BusOutputAsStruct=on
  qS : Inport  Port=2  BusOutputAsStruct=on
  Controls : Inport  Port=3  OutDataTypeStr=Bus: Controls_CMD_BUS  BusOutputAsStruct=on
  Add : Sum
  Add2 : Sum  Inputs=++++++++
  Add3 : Sum  Inputs=-+
  Bus Selector : BusSelector  OutputSignals=Alpha_A_R_B
  Bus Selector10 : BusSelector  OutputSignals=Actuators_CMD.DVTL
  Bus Selector2 : BusSelector  OutputSignals=Actuators_CMD.DAR
  Bus Selector3 : BusSelector  OutputSignals=Actuators_CMD.DVTR
  Bus Selector4 : BusSelector  OutputSignals=Beta_A_R_B
  Bus Selector5 : BusSelector  OutputSignals=Actuators_CMD.DAL
  Bus Selector6 : BusSelector  OutputSignals=VEL_K_R_ABS,ROT_K_R_B
  Bus Selector8 : BusSelector  OutputSignals=Actuators_CMD.DFR
  Cmq : Gain  Gain=AeroDerivatives.Cnr
  Constant : Constant  Value=Configuration.b
  Constant1 : Constant  Value=Configuration.b
  Divide : Product  Inputs=/*
  Gain10 : Gain  Gain=1/(2*Actuators.Pseudo.CAweight_De)
  Gain11 : Gain  Gain=1/(2*Actuators.Pseudo.CAweight_Dr)
  Gain12 : Gain  Gain=AeroDerivatives.CnDr
  Gain13 : Gain  Gain=AeroDerivatives.CnDf
  Gain14 : Gain  Gain=AeroDerivatives.CnDa
  Gain15 : Gain  Gain=AeroDerivatives.CnDa
  Gain6 : Gain
  Gain7 : Gain  Gain=AeroDerivatives.CnAlpha
  Gain8 : Gain  Gain=AeroDerivatives.CnBeta
  Gain9 : Gain  Gain=AeroDerivatives.CnDe
  Product2 : Product  Inputs=3
  Product5 : Product
  Saturation : Saturate  UpperLimit=inf  LowerLimit=10
  Selector : Selector  InputPortWidth=3  IndexOptions=Index vector (dialog)  Indices=[3]  OutputSizes=1
  Temporary1 : Gain  Gain=1/2
  Temporary2 : Gain  Gain=2
  Temporary4 : Gain  Gain=1/2
  MOMZ_A_R_W : Outport  Unit=N  PortDimensions=1
  wires:
  Bus Selector4/1 -> Gain8/1  "<Beta_A_R_B>"
  Gain14/1 -> Temporary4/1
  Gain8/1 -> Add2/2
  Gain10/1 -> Gain9/1
  qS/1 -> Product2/2
  Add2/1 -> Gain6/1
  Controls/1 -> Bus Selector8/1, Bus Selector2/1, Bus Selector5/1, Bus Selector3/1, Bus Selector10/1
  Bus Selector2/1 -> Gain14/1  "<DAR>"
  Gain15/1 -> Temporary1/1
  Gain6/1 -> Product2/3
  Bus Selector3/1 -> Add3/1, Add/1  "<DVTR>"
  Bus Selector/1 -> Gain7/1  "<Alpha_A_R_B>"
  Bus Selector8/1 -> Gain13/1  "<DFR>"
  Temporary1/1 -> Add2/7
  Temporary4/1 -> Add2/6
  Product2/1 -> MOMZ_A_R_W/1
  Bus Selector5/1 -> Gain15/1  "<DAL>"
  Gain7/1 -> Add2/1
  Gain13/1 -> Add2/5
  Gain11/1 -> Gain12/1
  Gain12/1 -> Add2/4
  Add3/1 -> Gain11/1
  Bus Selector10/1 -> Add3/2, Add/2  "<DVTL>"
  Add/1 -> Gain10/1
  Gain9/1 -> Add2/3
  Constant/1 -> Product2/1
  Temporary2/1 -> Saturation/1
  Selector/1 -> Product5/1
  Product5/1 -> Divide/2
  Bus Selector6/2 -> Selector/1  "<ROT_K_R_B>"
  Cmq/1 -> Add2/8
  Divide/1 -> Cmq/1
  Saturation/1 -> Divide/1
  Bus Selector6/1 -> Temporary2/1  "<VEL_K_R_ABS>"
  States/1 -> Bus Selector6/1, Bus Selector4/1, Bus Selector/1
  Constant1/1 -> Product5/2  "b"

== system Flight_Physics__ForStudent/Aerodynamics/Subsystem ==
  States : Inport
  Bus Selector : BusSelector  OutputSignals=POS_R_E,VEL_K_R_ABS
  Constant2 : Constant  Value=Configuration.S
  Gain : Gain  Gain=0.5
  ISA Atmosphere Model : aerolibatmos2/ISA Atmosphere Model  custom=off  g=9.80665  gamma=1.4  R=287.0531  L=0.0065  h_trop=11000  h_strat=20000  rho0=1.225  P0=101325  T0=288.15  h0=0
      settings: SourceProductName=Aerospace Blockset
  Math Function : Math  Operator=magnitude^2  SaturateOnIntegerOverflow=on
  Product : Product  Inputs=3
  Selector : Selector  InputPortWidth=3  IndexOptions=Index vector (dialog)  Indices=[3]  OutputSizes=1
  Terminator : Terminator
  Terminator2 : Terminator
  Terminator3 : Terminator
  qS : Outport
  wires:
  Selector/1 -> ISA Atmosphere Model/1
  ISA Atmosphere Model/1 -> Terminator2/1
  ISA Atmosphere Model/3 -> Terminator3/1
  States/1 -> Bus Selector/1
  Bus Selector/1 -> Selector/1  "<POS_R_E>"
  ISA Atmosphere Model/2 -> Terminator/1
  Constant2/1 -> Product/3
  ISA Atmosphere Model/4 -> Product/1
  Gain/1 -> Product/2
  Product/1 -> qS/1
  Math Function/1 -> Gain/1
  Bus Selector/2 -> Math Function/1  "<VEL_K_R_ABS>"

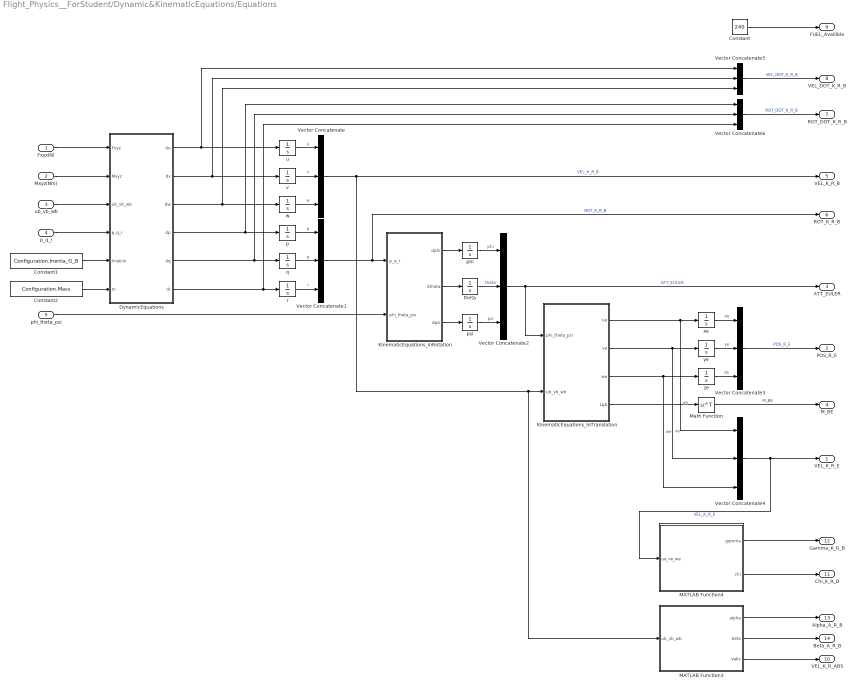
== system Flight_Physics__ForStudent/Dynamic&KinematlcEquations/Equations ==
  Fxyz(N) : Inport
  Mxyz(Nm) : Inport  Port=2
  ub_vb_wb : Inport  Port=3
  p_q_r : Inport  Port=4
  phi_theta_psi : Inport  Port=5
  Constant : Constant  Value=240
  Constant1 : Constant  Value=Configuration.Inertia_G_B
  Constant2 : Constant  Value=Configuration.Mass
  DynamicEquations : MATLAB Function  TreatAsAtomicUnit=on
  KinematicEquations_InRotation : MATLAB Function  TreatAsAtomicUnit=on
  KinematicEquations_InTranslation : MATLAB Function  TreatAsAtomicUnit=on
  MATLAB Function3 : MATLAB Function  TreatAsAtomicUnit=on
  MATLAB Function4 : MATLAB Function  TreatAsAtomicUnit=on
  Math Function : Math  Operator=transpose  SaturateOnIntegerOverflow=on
  Vector Concatenate{,1..6} (7 alike) : Concatenate  NumInputs=3
  p : Integrator  InitialCondition=Sim_Control.init(4,1)  ContinuousStateAttributes='p'
  phi : Integrator  InitialCondition=Sim_Control.init(3,1)  ContinuousStateAttributes='phi'
  psi : Integrator  InitialCondition=Sim_Control.init(3,3)  ContinuousStateAttributes='psi'
  q : Integrator  InitialCondition=Sim_Control.init(4,2)  ContinuousStateAttributes='q'
  r : Integrator  InitialCondition=Sim_Control.init(4,3)  ContinuousStateAttributes='r'
  theta : Integrator  InitialCondition=Sim_Control.init(3,2)  ContinuousStateAttributes='theta'
  u : Integrator  InitialCondition=Sim_Control.init(2,1)  ContinuousStateAttributes='ub'
  v : Integrator  InitialCondition=Sim_Control.init(2,2)  ContinuousStateAttributes='vb'
  w : Integrator  InitialCondition=Sim_Control.init(2,3)  ContinuousStateAttributes='wb'
  xe : Integrator  InitialCondition=Sim_Control.init(1,1)  ContinuousStateAttributes='xe'
  ye : Integrator  InitialCondition=Sim_Control.init(1,2)  ContinuousStateAttributes='ye'
  ze : Integrator  InitialCondition=Sim_Control.init(1,3)  ContinuousStateAttributes='ze'
  VEL_K_R_E : Outport
  POS_R_E : Outport  Port=2
  ATT_EULER : Outport  Port=3
  M_BE : Outport  Port=4
  VEL_K_R_B : Outport  Port=5
  ROT_K_R_B : Outport  Port=6
  ROT_DOT_K_R_B : Outport  Port=7
  VEL_DOT_K_R_B : Outport  Port=8
  FUEL_Availible : Outport  Port=9
  VEL_K_R_ABS : Outport  Port=10
  Chi_K_R_B : Outport  Port=11
  Gamma_K_R_B : Outport  Port=12
  Alpha_A_R_B : Outport  Port=13
  Beta_A_R_B : Outport  Port=14
  wires:
  DynamicEquations/5(dq) -> Vector Concatenate6/2, q/1
  w/1 -> Vector Concatenate/3  "w"
  u/1 -> Vector Concatenate/1  "u"
  DynamicEquations/3(dw) -> Vector Concatenate5/3, w/1
  KinematicEquations_InRotation/3(dpsi) -> psi/1
  KinematicEquations_InRotation/2(dtheta) -> theta/1
  Vector Concatenate2/1 -> ATT_EULER/1, KinematicEquations_InTranslation/1(phi_theta_psi)  "ATT_EULER"
  Vector Concatenate/1 -> VEL_K_R_B/1, KinematicEquations_InTranslation/2(ub_vb_wb), MATLAB Function3/1(ub_vb_wb)  "VEL_K_R_B"
  KinematicEquations_InTranslation/1(ue) -> Vector Concatenate4/1, xe/1  "ue"
  KinematicEquations_InTranslation/3(we) -> Vector Concatenate4/3, ze/1  "we"
  DynamicEquations/2(dv) -> Vector Concatenate5/2, v/1
  q/1 -> Vector Concatenate1/2  "q"
  r/1 -> Vector Concatenate1/3  "r"
  p/1 -> Vector Concatenate1/1  "p"
  KinematicEquations_InRotation/1(dphi) -> phi/1
  DynamicEquations/1(du) -> Vector Concatenate5/1, u/1
  v/1 -> Vector Concatenate/2  "v"
  DynamicEquations/6(dr) -> Vector Concatenate6/3, r/1
  psi/1 -> Vector Concatenate2/3  "psi"
  phi/1 -> Vector Concatenate2/1  "phi"
  Vector Concatenate1/1 -> ROT_K_R_B/1, KinematicEquations_InRotation/1(p_q_r)  "ROT_K_R_B"
  theta/1 -> Vector Concatenate2/2  "theta"
  ze/1 -> Vector Concatenate3/3  "ze"
  DynamicEquations/4(dp) -> Vector Concatenate6/1, p/1
  xe/1 -> Vector Concatenate3/1  "xe"
  KinematicEquations_InTranslation/2(ve) -> Vector Concatenate4/2, ye/1  "ve"
  ye/1 -> Vector Concatenate3/2  "ye"
  Fxyz(N)/1 -> DynamicEquations/1(Fxyz)
  Mxyz(Nm)/1 -> DynamicEquations/2(Mxyz)
  Vector Concatenate3/1 -> POS_R_E/1  "POS_R_E"
  Vector Concatenate4/1 -> VEL_K_R_E/1, MATLAB Function4/1(ue_ve_we)  "VEL_K_R_E"
  KinematicEquations_InTranslation/4(Lgb) -> Math Function/1
  Math Function/1 -> M_BE/1  "M_BE"
  Vector Concatenate6/1 -> ROT_DOT_K_R_B/1  "ROT_DOT_K_R_B"
  Vector Concatenate5/1 -> VEL_DOT_K_R_B/1  "VEL_DOT_K_R_B"
  Constant/1 -> FUEL_Availible/1
  MATLAB Function3/1(alpha) -> Alpha_A_R_B/1
  MATLAB Function3/2(beta) -> Beta_A_R_B/1
  MATLAB Function3/3(Vabs) -> VEL_K_R_ABS/1
  MATLAB Function4/1(gamma) -> Gamma_K_R_B/1
  MATLAB Function4/2(chi) -> Chi_K_R_B/1
  ub_vb_wb/1 -> DynamicEquations/3(ub_vb_wb)
  p_q_r/1 -> DynamicEquations/4(p_q_r)
  Constant1/1 -> DynamicEquations/5(Imatrix)
  Constant2/1 -> DynamicEquations/6(m)
  phi_theta_psi/1 -> KinematicEquations_InRotation/2(phi_theta_psi)

== system Flight_Physics__ForStudent/Engines/Subsystem ==
  note: [cosP  0     sinP
      |  0        1     0
      | -sinP   0     cosP ]
  Phi_rad : Inport  Unit=rad  PortDimensions=[1,1]
  Constant : Constant
  Constant1 : Constant  Value=0
  Gain1 : Gain  Gain=-1
  Saturation1 : Saturate  UpperLimit=4*pi  LowerLimit=-4*pi
  Trigonometric Function : Trigonometry  Operator=sincos  NumberOfIterations=15
  Vector Concatenate : Concatenate  NumInputs=3
  Vector Concatenate1 : Concatenate  NumInputs=3
  Vector Concatenate2 : Concatenate  NumInputs=3
  Vector Concatenate3 : Concatenate  NumInputs=3  Mode=Multidimensional array  ConcatenateDimension=2
  M_B_Phi : Outport  PortDimensions=[3,3]
  wires:
  Constant1/1 -> Vector Concatenate/2, Vector Concatenate1/1, Vector Concatenate1/3, Vector Concatenate2/2
  Trigonometric Function/2 -> Vector Concatenate/1, Vector Concatenate2/3
  Constant/1 -> Vector Concatenate1/2
  Vector Concatenate/1 -> Vector Concatenate3/1
  Gain1/1 -> Vector Concatenate/3
  Trigonometric Function/1 -> Gain1/1, Vector Concatenate2/1
  Vector Concatenate2/1 -> Vector Concatenate3/3
  Saturation1/1 -> Trigonometric Function/1
  Phi_rad/1 -> Saturation1/1
  Vector Concatenate3/1 -> M_B_Phi/1
  Vector Concatenate1/1 -> Vector Concatenate3/2

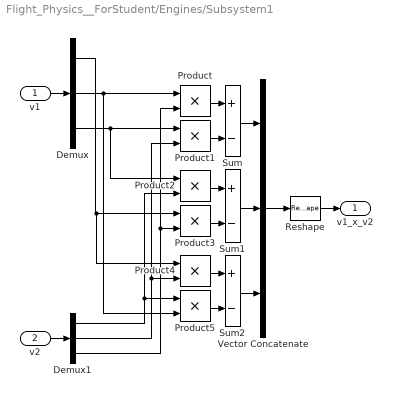
== system Flight_Physics__ForStudent/Engines/Subsystem1 ==
  v1 : Inport  PortDimensions=[3,1]
  v2 : Inport  Port=2  PortDimensions=[3,1]
  Demux : Demux  Outputs=3
  Demux1 : Demux  Outputs=3
  Product{,1..5} (6 alike) : Product
  Reshape : Reshape  OutputDimensionality=Column vector (2-D)  OutputDimensions=1
  Sum : Sum  Inputs=+-
  Sum1 : Sum  Inputs=+-
  Sum2 : Sum  Inputs=+-
  Vector Concatenate : Concatenate  NumInputs=3
  v1_x_v2 : Outport  PortDimensions=[3,1]
  wires:
  v1/1 -> Demux/1
  Product4/1 -> Sum2/1
  v2/1 -> Demux1/1
  Demux/2 -> Product/1, Product5/2
  Vector Concatenate/1 -> Reshape/1
  Reshape/1 -> v1_x_v2/1
  Sum1/1 -> Vector Concatenate/2
  Demux1/1 -> Product2/2, Product5/1
  Product2/1 -> Sum1/1
  Demux1/2 -> Product1/2, Product4/2
  Product1/1 -> Sum/2
  Demux/1 -> Product3/1, Product4/1
  Product5/1 -> Sum2/2
  Demux1/3 -> Product/2, Product3/2
  Product3/1 -> Sum1/2
  Sum2/1 -> Vector Concatenate/3
  Product/1 -> Sum/1
  Demux/3 -> Product2/1, Product1/1
  Sum/1 -> Vector Concatenate/1

== system Flight_Physics__ForStudent/FOR_MOM_Summation/Subsystem ==
  v1 : Inport  PortDimensions=[3,1]
  v2 : Inport  Port=2  PortDimensions=[3,1]
  Demux : Demux  Outputs=3
  Demux1 : Demux  Outputs=3
  Product{,1..5} (6 alike) : Product
  Reshape : Reshape  OutputDimensionality=Column vector (2-D)  OutputDimensions=1
  Sum : Sum  Inputs=+-
  Sum1 : Sum  Inputs=+-
  Sum2 : Sum  Inputs=+-
  Vector Concatenate : Concatenate  NumInputs=3
  v1_x_v2 : Outport  PortDimensions=[3,1]
  wires:
  Vector Concatenate/1 -> Reshape/1
  Sum/1 -> Vector Concatenate/1
  v2/1 -> Demux1/1
  Product/1 -> Sum/1
  Product3/1 -> Sum1/2
  Product2/1 -> Sum1/1
  Reshape/1 -> v1_x_v2/1
  Sum1/1 -> Vector Concatenate/2
  Sum2/1 -> Vector Concatenate/3
  Demux1/3 -> Product/2, Product3/2
  Demux/3 -> Product2/1, Product1/1
  Demux/2 -> Product/1, Product5/2
  Demux1/2 -> Product1/2, Product4/2
  Product5/1 -> Sum2/2
  v1/1 -> Demux/1
  Demux1/1 -> Product2/2, Product5/1
  Product1/1 -> Sum/2
  Demux/1 -> Product3/1, Product4/1
  Product4/1 -> Sum2/1

== system Flight_Physics__ForStudent/FOR_MOM_Summation/Subsystem1 ==
  V : Inport
  Math Function : Math  Operator=magnitude^2  SaturateOnIntegerOverflow=on
  Sqrt : Sqrt  SaturateOnIntegerOverflow=on
  Sum : Sum  Inputs=+
  ||V|| : Outport
  wires:
  Sqrt/1 -> ||V||/1
  Sum/1 -> Sqrt/1
  Math Function/1 -> Sum/1
  V/1 -> Math Function/1

== matlab function Flight_Physics__ForStudent/Dynamic&KinematlcEquations/Equations/KinematicEquations_InRotation ==
  data: p_q_r input; dphi output; phi_theta_psi input; dtheta output; dpsi output
function [dphi, dtheta, dpsi] = fcn(p_q_r, phi_theta_psi)
p = p_q_r(1);
q = p_q_r(2);
r = p_q_r(3);
phi = phi_theta_psi(1);
theta = phi_theta_psi(2);



%%%%%%%%%%%%%%%%%%%%%%%%%%%%%%%%%%%%%%%%%%%%%%%%%%%%%%%%%%%%%%%%%%%%%%%%%%%
% 根据式（4.3）写出正确形式的建模公式
% 注意：
%   正确公式需要对式（4.3）做一定的变换才能得到，请***自行推导***
%   等号左边为微分量，作为函数输出，等号右边为已知量，即函数输入
%   等号右边请使用前面定义好的变量，如p，q，r等

dphi = 0;%将0替换为正确的公式
dtheta = 0;%将0替换为正确的公式
dpsi = 0;%将0替换为正确的公式


%   公式补全后快捷键Ctrl+S保存
%%%%%%%%%%%%%%%%%%%%%%%%%%%%%%%%%%%%%%%%%%%%%%%%%%%%%%%%%%%%%%%%%%%%%%%%%%%


end

== matlab function Flight_Physics__ForStudent/Dynamic&KinematlcEquations/Equations/DynamicEquations ==
  data: Fxyz input; du output; Mxyz input; ub_vb_wb input; p_q_r input; Imatrix input; m input; dv output; dw output; dp output; dq output; dr output
function [du, dv, dw, dp, dq, dr] = fcn(Fxyz, Mxyz, ub_vb_wb, p_q_r, Imatrix, m)
Fx = Fxyz(1);
Fy = Fxyz(2);
Fz = Fxyz(3);
Mx = Mxyz(1);
My = Mxyz(2);
Mz = Mxyz(3);
u = ub_vb_wb(1);
v = ub_vb_wb(2);
w = ub_vb_wb(3);
p = p_q_r(1);
q = p_q_r(2);
r = p_q_r(3);
Ix = Imatrix(1,1);
Iy = Imatrix(2,2);
Iz = Imatrix(3,3);
Izx = Imatrix(1,3);

%%%%%%%%%%%%%%%%%%%%%%%%%%%%%%%%%%%%%%%%%%%%%%%%%%%%%%%%%%%%%%%%%%%%%%%%%%%
% 根据式（4.2）写出正确形式的建模公式
% 注意：
%   正确公式需要对式（4.2）做一定的变换才能得到，请***自行推导***
%   等号左边为微分量，作为函数输出，等号右边为已知量，即函数输入
%   等号右边请使用前面定义好的变量，如Mx，u，p，Izx等


du=0;%将0替换为正确的公式
dv=0;%将0替换为正确的公式
dw=0;%将0替换为正确的公式
dp=0;%将0替换为正确的公式
dq=0;%将0替换为正确的公式
dr=0;%将0替换为正确的公式


%   公式补全后快捷键Ctrl+S保存
%%%%%%%%%%%%%%%%%%%%%%%%%%%%%%%%%%%%%%%%%%%%%%%%%%%%%%%%%%%%%%%%%%%%%%%%%%%

end

== matlab function Flight_Physics__ForStudent/Dynamic&KinematlcEquations/Equations/KinematicEquations_InTranslation ==
  data: phi_theta_psi input; ub_vb_wb input; ue output; ve output; we output; Lgb output
function [ue, ve, we, Lgb] = fcn(phi_theta_psi, ub_vb_wb)
phi = phi_theta_psi(1);
theta = phi_theta_psi(2);
psi = phi_theta_psi(3);


Lgb=...
  [ cos(psi)*cos(theta), cos(psi)*sin(phi)*sin(theta) - cos(phi)*sin(psi), sin(phi)*sin(psi) + cos(phi)*cos(psi)*sin(theta);
    cos(theta)*sin(psi), cos(phi)*cos(psi) + sin(phi)*sin(psi)*sin(theta), cos(phi)*sin(psi)*sin(theta) - cos(psi)*sin(phi);
          -sin(theta),                        cos(theta)*sin(phi),                        cos(phi)*cos(theta)];
 
ue_ve_we=Lgb*ub_vb_wb;
ue = ue_ve_we(1);
ve = ue_ve_we(2);
we = ue_ve_we(3);
end

== matlab function Flight_Physics__ForStudent/Dynamic&KinematlcEquations/Equations/MATLAB Function4 ==
  data: ue_ve_we input; gamma output; chi output
function [gamma, chi] = fcn(ue_ve_we)
u = ue_ve_we(1);
v = ue_ve_we(2);
w = ue_ve_we(3);

Vabs = sqrt(u*u+v*v+w*w);
if Vabs<0.01
    Vabs_lim = 0.01;
else
    Vabs_lim = Vabs;
end
gamma = asin(w/Vabs_lim);
chi = atan(v/u);
if chi<0
    chi = chi+2*pi;
end


end

== matlab function Flight_Physics__ForStudent/Dynamic&KinematlcEquations/Equations/MATLAB Function3 ==
  data: ub_vb_wb input; alpha output; beta output; Vabs output
function [alpha, beta, Vabs] = fcn(ub_vb_wb)
u = ub_vb_wb(1);
v = ub_vb_wb(2);
w = ub_vb_wb(3);

alpha = atan(w/u);
Vabs = sqrt(u*u+v*v+w*w);
if Vabs<0.01
    Vabs = 0.01;
end
beta = asin(v/Vabs);

end
